simulink model "Hybrid_P2_Parallel_ETE"  (R2017b)
settings: Solver=FixedStepAuto  StartTime=0.0  StopTime=length(Speed)  FixedStep=0.01  MaxStep=0.01  RelTol=1e-3  EnableMultiTasking=on
PostLoadFcn:
  | , if any(exist('dsrtsu_mdlpostloadfcn', 'file') == [2, 3, 6]), try dsrtsu_mdlpostloadfcn('Execute', bdroot); catch fprintf('Error in PostLoadFcn (dsrtsu_mdlpostloadfcn) for model "%s":\n %s\n', bdroot, lasterr); end, end,
undefined symbols (not defined in the file): Actuators, APP1_OOR, APP2_OOR, APP_Mismatch, Brk_Flt, cal, ClutchEngag, CycLength, CycNmb, DiscIntNeverNeededParam, eng, Engine, EngOverTemp, ENGTRQ_MSMCH_Degraded_CP, ENGTRQ_MSMCH_ErrCritical_CP, ENGTRQ_MSMCH_LimpHome_CP, EngTrqMismatch, ess, ESSOverTemp, gb, Gearbox, KeyPos_Flt, lib_Actuators, lib_EMachine_2017a, lib_Sensors_2017a, Loss, LossCAN, Machine, MCUOverTemp, mot, MotDirMismatch, MotOverTemp, MotTrqMismatch, PRNDL_Flt, Ratio, RegenFault, Scope_new, Scopes1, Sensors, Spd, StopIndex, t_amb, time, tloop
libraries: simulink x117, EC2_libraries x9, powerlib_meascontrol x2, CalculationGallon x1, lib_Chassis x1, lib_DCDC x1, lib_Differential x1, lib_HVESS x1, lib_Engine x1, lib_OBC x1, lib_Transmission x1, Transmission_Validation x1
(part 9 of 10)

== system Hybrid_P2_Parallel_ETE/Controller_with_Transmission_Manager1/HSC/Powertrain Manager/HV Manager1/DCDC Manager/Override_Voltage ==
  In1 : Inport
  Switch : Switch  Criteria=u2 > Threshold
  VoltageHVOvrrdSW : Constant  Value=0
  voltageHVOvrrdVal : Constant  Value=0
  Out1 : Outport
  wires:
  voltageHVOvrrdVal/1 -> Switch/1
  VoltageHVOvrrdSW/1 -> Switch/2
  In1/1 -> Switch/3
  Switch/1 -> Out1/1  "DC_mode"

== system Hybrid_P2_Parallel_ETE/Controller_with_Transmission_Manager1/HSC/Powertrain Manager/HV Manager1/DCDC Manager/Override_VoltageLV ==
  In1 : Inport
  Switch : Switch  Criteria=u2 > Threshold
  VoltageLVOvrrdSW : Constant  Value=0
  VoltageLVOvrrdVAL : Constant  Value=14
  Out1 : Outport
  wires:
  VoltageLVOvrrdVAL/1 -> Switch/1
  VoltageLVOvrrdSW/1 -> Switch/2
  In1/1 -> Switch/3
  Switch/1 -> Out1/1  "DC_mode"

== system Hybrid_P2_Parallel_ETE/Controller_with_Transmission_Manager1/HSC/Powertrain Manager/HV Manager1/DCDC Manager/Override_mode ==
  In1 : Inport
  DCDCOVrrdSwitch : Constant  Value=0
  DCDCOVrrdVal : Constant  Value=0
  Switch : Switch  Criteria=u2 > Threshold
  Out1 : Outport
  wires:
  Switch/1 -> Out1/1  "DC_mode"
  In1/1 -> Switch/3
  DCDCOVrrdSwitch/1 -> Switch/2
  DCDCOVrrdVal/1 -> Switch/1

== system Hybrid_P2_Parallel_ETE/Controller_with_Transmission_Manager1/HSC/Powertrain Manager/Torque Distribution1/AxlTrq_to_EngTrq2/Ratio Filter ==
  Ratio : Inport
  Abs : Abs
  Compare To Zero : simulink/Logic and Bit Operations/Compare To Zero  relop===  OutDataTypeStr=boolean
  Constant : Constant  Value=cal.Time.TrnsOvrllEstTrqRatioSwitch
  Mature_Delay : EC2_libraries/Mature_Delay
  Memory1 : Memory  InitialCondition=1
  Switch1 : Switch  Threshold=1
  Switch2 : Switch  Threshold=1
  Filtered_Ratio : Outport
  wires:
  Ratio/1 -> Compare To Zero/1, Abs/1
  Compare To Zero/1 -> Mature_Delay/1, Switch2/2
  Abs/1 -> Switch1/1, Switch2/3
  Switch1/1 -> Switch2/1
  Constant/1 -> Mature_Delay/2
  Mature_Delay/1 -> Switch1/2
  Memory1/1 -> Switch1/3
  Switch2/1 -> Filtered_Ratio/1, Memory1/1  "gear_ratio"

== system Hybrid_P2_Parallel_ETE/Controller_with_Transmission_Manager1/HSC/Powertrain Manager/Torque Distribution1/AxlTrq_to_MotTrq/AxlTrq_to_MtrTrq2 ==
  note: //From motor axle torque to motor torque//
  In1 : Inport
  Compare To Constant : simulink/Logic and Bit Operations/Compare To Constant  relop===  const=0  OutDataTypeStr=boolean
  Constant1 : Constant  Value=max(gb.plant.init.ratio.map)
  Constant5 : Constant  Value=fd.plant.init.ratio
  Divide : Product  Inputs=*//
  Rate Limiter1 : RateLimiter  Commented=on  RisingSlewLimit=20000  FallingSlewLimit=-20000
  Ratio Filter : Subsystem
  Switch : Switch  Criteria=u2 > Threshold
  MtrTrqCmd : Outport
  wires:
  In1/1 -> Divide/1  "MotAxlTrq"
  Constant5/1 -> Divide/2
  [TransRatio] -> Ratio Filter/1(Ratio)
  Compare To Constant/1 -> Switch/2
  Constant1/1 -> Switch/1
  Divide/1 -> MtrTrqCmd/1  "Axl2MotTrq"
  Switch/1 -> Divide/3  "TrnsFilRatio"
  Ratio Filter/1(Filtered_Ratio) -> Switch/3, Compare To Constant/1  "FilteredRatio"

== system Hybrid_P2_Parallel_ETE/Controller_with_Transmission_Manager1/HSC/Powertrain Manager/Torque Distribution1/AxlTrq_to_MotTrq/electric machine filter ==
  trq : Inport
  Interval Test : simulink/Logic and Bit Operations/Interval Test  IntervalClosedRight=on  uplimit=0.02  IntervalClosedLeft=on  lowlimit=-0.02  OutDataTypeStr=boolean
  Switch : Switch  Threshold=0.5
  electric machine time response : TransferFcn  Denominator=[mot.plant.init.time_response 1]
  filtered : Outport
  wires:
  electric machine time response/1 -> Switch/3
  Interval Test/1 -> Switch/2
  trq/1 -> Interval Test/1, electric machine time response/1, Switch/1
  Switch/1 -> filtered/1  "MotTrqFil"

== system Hybrid_P2_Parallel_ETE/Controller_with_Transmission_Manager1/HSC/Powertrain Manager/Torque Distribution1/Hood_Status/Close_Voltage ==
  DC_Voltage : Inport
  Constant : Constant  Value=2.3
  Constant1 : Constant  Value=3.03
  Divide : Product  Inputs=*/*
  Out1 : Outport
  wires:
  Divide/1 -> Out1/1
  Constant/1 -> Divide/1
  Constant1/1 -> Divide/2
  DC_Voltage/1 -> Divide/3

== system Hybrid_P2_Parallel_ETE/Controller_with_Transmission_Manager1/HSC/Powertrain Manager/Torque Distribution1/Hood_Status/Open_Voltage ==
  DC_Voltage : Inport
  Constant2 : Constant  Value=0.73
  Constant3 : Constant  Value=3.03
  Divide1 : Product  Inputs=*/*
  Out1 : Outport
  wires:
  Divide1/1 -> Out1/1
  Constant2/1 -> Divide1/1
  DC_Voltage/1 -> Divide1/3
  Constant3/1 -> Divide1/2

== system Hybrid_P2_Parallel_ETE/Controller_with_Transmission_Manager1/HSC/Powertrain Manager/Torque Distribution1/IdealMotTrq/MotTrq2AxlTrq ==
  In1 : Inport
  Compare To Constant : simulink/Logic and Bit Operations/Compare To Constant  relop===  const=0  OutDataTypeStr=boolean
  Constant1 : Constant  Value=max(gb.plant.init.ratio.map)
  Constant2 : Constant  Value=fd.plant.init.ratio
  Divide1 : Product  Inputs=***
  Ratio Filter : Subsystem
  Switch : Switch  Criteria=u2 > Threshold
  Out1 : Outport
  wires:
  Ratio Filter/1(Filtered_Ratio) -> Compare To Constant/1, Switch/3  "FilteredRatio"
  Switch/1 -> Divide1/1  "TrnsFilRatio"
  Constant1/1 -> Switch/1
  Compare To Constant/1 -> Switch/2
  Constant2/1 -> Divide1/2
  [TransRatio] -> Ratio Filter/1(Ratio)
  In1/1 -> Divide1/3
  Divide1/1 -> Out1/1  "P"

== system Hybrid_P2_Parallel_ETE/Controller_with_Transmission_Manager1/HSC/Powertrain Manager/Torque Distribution1/IdealMotTrq/Subsystem ==
  Setpoint : Inport
  Actual : Inport  Port=2
  Add : Sum  Inputs=+-
  Add2 : Sum
  IdleTorqueVal : Constant  Value=7
  Kp : Constant  Value=0.2
  Product : Product
  Out1 : Outport
  wires:
  Actual/1 -> Add/2
  Setpoint/1 -> Add/1
  Kp/1 -> Product/2
  IdleTorqueVal/1 -> Add2/2
  Add2/1 -> Out1/1
  Add/1 -> Product/1
  Product/1 -> Add2/1

== system Hybrid_P2_Parallel_ETE/Controller_with_Transmission_Manager1/HSC/Powertrain Manager/Torque Distribution1/Supervisory  Control  Logic1/VehReady.CD_Mode.Drive_mode.MotTrqCalc2/Motor idle torque1 ==
  In1 : Inport
  Constant2 : Constant  Value=fd.plant.init.ratio
  Constant3 : Constant  Value=0
  Divide1 : Product  Inputs=***
  Out1 : Outport
  wires:
  In1/1 -> Divide1/1
  Constant2/1 -> Divide1/2
  Constant3/1 -> Divide1/3
  Divide1/1 -> Out1/1  "P"

== system Hybrid_P2_Parallel_ETE/Controller_with_Transmission_Manager1/HSC/Powertrain Manager/Torque Distribution1/Supervisory  Control  Logic1/VehReady.Eng_Charging_Stat.EngTrqCalc/Multiply by Zero fix ==
  In1 : Inport
  Compare To Constant : simulink/Logic and Bit Operations/Compare To Constant  relop===  const=0  OutDataTypeStr=boolean
  Constant5 : Constant  Value=max(gb.plant.init.ratio.map)
  Ratio Filter : Subsystem
  Switch : Switch  Criteria=u2 > Threshold
  Out1 : Outport
  wires:
  In1/1 -> Ratio Filter/1(Ratio)
  Compare To Constant/1 -> Switch/2
  Constant5/1 -> Switch/1
  Switch/1 -> Out1/1  "TrnsFilRatio"
  Ratio Filter/1(Filtered_Ratio) -> Switch/3, Compare To Constant/1  "FilteredRatio"

== system Hybrid_P2_Parallel_ETE/Camaro Plant Model/E-Machine/IMG Plant/Electric Machine/Thermal1/MotInv_loop/MCUOverTemp Fault ==
  In1 : Inport
  Gain : Gain  Gain=3
  Switch : Switch  Threshold=1
  Out1 : Outport
  wires:
  Switch/1 -> Out1/1
  Gain/1 -> Switch/1
  [MCUOverTemp] -> Switch/2
  In1/1 -> Gain/1, Switch/3

== system Hybrid_P2_Parallel_ETE/Camaro Plant Model/E-Machine/IMG Plant/Electric Machine/Thermal1/MotInv_loop/MotorOverTempFault ==
  In1 : Inport
  Gain : Gain  Gain=2
  Memory : Memory
  Switch1 : Switch  Threshold=1
  Out1 : Outport
  wires:
  Switch1/1 -> Out1/1
  Gain/1 -> Switch1/1
  [MotOverTemp] -> Switch1/2
  In1/1 -> Switch1/3, Memory/1
  Memory/1 -> Gain/1

== system Hybrid_P2_Parallel_ETE/Camaro Plant Model/E-Machine/IMG Plant/Electric Machine/Thermal1/Motor Thermal/Lower Limit ==
  In1 : Inport
  Constant3 : Constant  Value=Lolimit
  MinMax : MinMax  Function=max  Inputs=2
  Out1 : Outport
  wires:
  MinMax/1 -> Out1/1
  Constant3/1 -> MinMax/2
  In1/1 -> MinMax/1

== system Hybrid_P2_Parallel_ETE/Camaro Plant Model/E-Machine/Soft MCU/Torque Calculation1/max torque /Heat index/Divide ==
  note: Take care of
      | division by 0
  numerator : Inport
  denominator : Inport  Port=2
  Fcn : Fcn  Expr=u[1] / ( u[2] + eps*(u[2]==0) )
  Mux : Mux  Inputs=2
  quotient : Outport
  wires:
  denominator/1 -> Mux/2
  Fcn/1 -> quotient/1
  numerator/1 -> Mux/1
  Mux/1 -> Fcn/1

== system Hybrid_P2_Parallel_ETE/Camaro Plant Model/E-Machine/Soft MCU/Torque Calculation2/max torque /Heat index/Divide ==
  note: Take care of
      | division by 0
  numerator : Inport
  denominator : Inport  Port=2
  Fcn : Fcn  Expr=u[1] / ( u[2] + eps*(u[2]==0) )
  Mux : Mux  Inputs=2
  quotient : Outport
  wires:
  denominator/1 -> Mux/2
  Fcn/1 -> quotient/1
  numerator/1 -> Mux/1
  Mux/1 -> Fcn/1

== system Hybrid_P2_Parallel_ETE/Camaro Plant Model/Transmission/Transmission Plant/Gearbox/Speed Calculation/P//N/Subsystem2 ==
  In1 : Inport
  In2 : Inport  Port=2
  Fcn : Fcn  Expr=u[1]/(u[2]+eps)*(u[2]!=0)
  Mux : Mux  Inputs=2
  Out1 : Outport
  wires:
  In2/1 -> Mux/2
  Fcn/1 -> Out1/1
  In1/1 -> Mux/1
  Mux/1 -> Fcn/1

== system Hybrid_P2_Parallel_ETE/Camaro Plant Model/Transmission/Transmission Plant/Gearbox/Speed Calculation/P//N/input shaft free wheeling losses ==
  input shaft speed : Inport
  Constant1 : Constant  Value=0
  Fcn1 : Fcn  Expr=u==0
  Gain1 : Gain  Gain=0.15  SaturateOnIntegerOverflow=on  OutDataTypeStr=Inherit: Same as input  ParamDataTypeStr=Inherit: Same as input
  Switch2 : Switch  Threshold=0.5  SaturateOnIntegerOverflow=on  InputSameDT=on
  input shaft decel : Outport
  wires:
  Constant1/1 -> Switch2/1
  Switch2/1 -> Gain1/1
  Gain1/1 -> input shaft decel/1
  Fcn1/1 -> Switch2/2
  input shaft speed/1 -> Fcn1/1, Switch2/3

== system Hybrid_P2_Parallel_ETE/Camaro Plant Model/Transmission/Transmission Plant/Gearbox/Speed Calculation/R//D/S-R Flip-Flop ==
  S : Inport
  R : Inport  Port=2
  Demux : Demux  Outputs=2
  Logic : CombinatorialLogic  TruthTable=[0 1;0 1;1 0;0 1;1 0;0 1;1 0;1 0]
  Memory : Memory  InitialCondition=initial_condition  InheritSampleTime=on
  Mux : Mux  Inputs=3
  Q : Outport  InitialOutput=0
  !Q : Outport  Port=2  InitialOutput=1
  wires:
  Mux/1 -> Logic/1
  Logic/1 -> Demux/1
  Demux/2 -> !Q/1
  Demux/1 -> Q/1, Memory/1
  Memory/1 -> Mux/1
  S/1 -> Mux/2
  R/1 -> Mux/3

== system Hybrid_P2_Parallel_ETE/Controller_with_Transmission_Manager1/HSC/Camaro Fault Detection/Signal Diagnostic/ESS Signal Diagnostic/ESS SOC Validity Check/essSOCValidity_Check ==
  In1 : Inport
  Above Normal Operation : simulink/Logic and Bit Operations/Compare To Constant  relop===  const=3  OutDataTypeStr=boolean
  Below Normal Operation : simulink/Logic and Bit Operations/Compare To Constant  relop===  const=0  OutDataTypeStr=boolean
  Logical Operator : Logic  Operator=OR  AllPortsSameDT=off  OutDataTypeStr=boolean
  Logical Operator1 : Logic  Operator=NOT  AllPortsSameDT=off  OutDataTypeStr=boolean
  Out1 : Outport
  wires:
  In1/1 -> Above Normal Operation/1, Below Normal Operation/1
  Logical Operator/1 -> Logical Operator1/1
  Below Normal Operation/1 -> Logical Operator/1
  Above Normal Operation/1 -> Logical Operator/2
  Logical Operator1/1 -> Out1/1

== system Hybrid_P2_Parallel_ETE/Controller_with_Transmission_Manager1/HSC/Camaro Fault Detection/Signal Diagnostic/ESS Signal Diagnostic/ESS Temp Validity Check/essTsignalValidity_Check ==
  In1 : Inport
  Above Normal Operation : simulink/Logic and Bit Operations/Compare To Constant  relop===  const=4  OutDataTypeStr=boolean
  Below Normal Operation : simulink/Logic and Bit Operations/Compare To Constant  relop===  const=0  OutDataTypeStr=boolean
  Logical Operator : Logic  Operator=OR  AllPortsSameDT=off  OutDataTypeStr=boolean
  Logical Operator1 : Logic  Operator=NOT  AllPortsSameDT=off  OutDataTypeStr=boolean
  Out1 : Outport
  wires:
  Logical Operator1/1 -> Out1/1
  Above Normal Operation/1 -> Logical Operator/2
  Below Normal Operation/1 -> Logical Operator/1
  Logical Operator/1 -> Logical Operator1/1
  In1/1 -> Below Normal Operation/1, Above Normal Operation/1

== system Hybrid_P2_Parallel_ETE/Controller_with_Transmission_Manager1/HSC/Driver_Requests/APP_BPP to DrvIntndAxlTrq2/Post Driver Intnded Axle Torque/Brake Command/Latch ==
  Input : Inport
  Reset : Inport  Port=2
  Logical Operator1 : Logic  Operator=NOT  AllPortsSameDT=off  OutDataTypeStr=boolean
  Logical Operator2 : Logic  AllPortsSameDT=off  OutDataTypeStr=boolean
  Logical Operator3 : Logic  Operator=OR  AllPortsSameDT=off  OutDataTypeStr=boolean
  Memory1 : Memory
  Out1 : Outport
  wires:
  Logical Operator2/1 -> Logical Operator3/2
  Reset/1 -> Logical Operator1/1
  Memory1/1 -> Logical Operator2/2
  Logical Operator3/1 -> Out1/1, Memory1/1
  Logical Operator1/1 -> Logical Operator2/1
  Input/1 -> Logical Operator3/1

== system Hybrid_P2_Parallel_ETE/Controller_with_Transmission_Manager1/HSC/Driver_Requests/APP_BPP to DrvIntndAxlTrq2/Post Driver Intnded Axle Torque/Driver Intended Axle Torque/Ratio Filter ==
  Ratio : Inport
  Abs : Abs
  Compare To Zero : simulink/Logic and Bit Operations/Compare To Zero  relop===  OutDataTypeStr=boolean
  Constant : Constant  Value=cal.Time.TrnsOvrllEstTrqRatioSwitch
  Mature_Delay : EC2_libraries/Mature_Delay
  Memory1 : Memory  InitialCondition=1
  Switch1 : Switch  Threshold=1
  Switch2 : Switch  Threshold=1
  Filtered_Ratio : Outport
  wires:
  Ratio/1 -> Compare To Zero/1, Abs/1
  Compare To Zero/1 -> Mature_Delay/1, Switch2/2
  Abs/1 -> Switch1/1, Switch2/3
  Switch1/1 -> Switch2/1
  Constant/1 -> Mature_Delay/2
  Mature_Delay/1 -> Switch1/2
  Memory1/1 -> Switch1/3
  Switch2/1 -> Filtered_Ratio/1, Memory1/1  "gear_ratio"

== system Hybrid_P2_Parallel_ETE/Controller_with_Transmission_Manager1/HSC/Powertrain Manager/HV Manager1/BMS_Manager/Isolation Fault Calculation/Resistance_Measurement ==
  In1 : Inport
  In2 : Inport  Port=2
  Enable : EnablePort
  Add : Sum
  ISOfault : Constant
  ISOmultiplier : Constant  Value=256
  ISOnofault : Constant  Value=0
  Minimum Allowed Isolation Resistance : Switch  Criteria=u2 > Threshold  Threshold=500000
  Product : Product
  Product1 : Product
  Resistance Adjustment : Constant  Value=1000
  IsoFault : Outport
  wires:
  Minimum Allowed Isolation Resistance/1 -> IsoFault/1  "IsoFault"
  ISOnofault/1 -> Minimum Allowed Isolation Resistance/1
  Resistance Adjustment/1 -> Product1/2
  Product1/1 -> Minimum Allowed Isolation Resistance/2
  ISOfault/1 -> Minimum Allowed Isolation Resistance/3
  Add/1 -> Product1/1
  Product/1 -> Add/1
  In2/1 -> Add/2
  In1/1 -> Product/1
  ISOmultiplier/1 -> Product/2

== system Hybrid_P2_Parallel_ETE/Controller_with_Transmission_Manager1/HSC/Powertrain Manager/Torque Distribution1/AxlTrq_to_MotTrq/AxlTrq_to_MtrTrq2/Ratio Filter ==
  Ratio : Inport
  Abs : Abs
  Compare To Zero : simulink/Logic and Bit Operations/Compare To Zero  relop===  OutDataTypeStr=boolean
  Constant : Constant  Value=cal.Time.TrnsOvrllEstTrqRatioSwitch
  Mature_Delay : EC2_libraries/Mature_Delay
  Memory1 : Memory  InitialCondition=1
  Switch1 : Switch  Threshold=1
  Switch2 : Switch  Threshold=1
  Filtered_Ratio : Outport
  wires:
  Ratio/1 -> Compare To Zero/1, Abs/1
  Compare To Zero/1 -> Mature_Delay/1, Switch2/2
  Abs/1 -> Switch1/1, Switch2/3
  Switch1/1 -> Switch2/1
  Constant/1 -> Mature_Delay/2
  Mature_Delay/1 -> Switch1/2
  Memory1/1 -> Switch1/3
  Switch2/1 -> Filtered_Ratio/1, Memory1/1  "gear_ratio"

== system Hybrid_P2_Parallel_ETE/Controller_with_Transmission_Manager1/HSC/Powertrain Manager/Torque Distribution1/IdealMotTrq/MotTrq2AxlTrq/Ratio Filter ==
  Ratio : Inport
  Abs : Abs
  Compare To Zero : simulink/Logic and Bit Operations/Compare To Zero  relop===  OutDataTypeStr=boolean
  Constant : Constant  Value=cal.Time.TrnsOvrllEstTrqRatioSwitch
  Mature_Delay : EC2_libraries/Mature_Delay
  Memory1 : Memory  InitialCondition=1
  Switch1 : Switch  Threshold=1
  Switch2 : Switch  Threshold=1
  Filtered_Ratio : Outport
  wires:
  Switch2/1 -> Memory1/1, Filtered_Ratio/1  "gear_ratio"
  Memory1/1 -> Switch1/3
  Mature_Delay/1 -> Switch1/2
  Constant/1 -> Mature_Delay/2
  Switch1/1 -> Switch2/1
  Abs/1 -> Switch2/3, Switch1/1
  Compare To Zero/1 -> Switch2/2, Mature_Delay/1
  Ratio/1 -> Abs/1, Compare To Zero/1

== system Hybrid_P2_Parallel_ETE/Controller_with_Transmission_Manager1/HSC/Powertrain Manager/Torque Distribution1/Supervisory  Control  Logic1/VehReady.Eng_Charging_Stat.EngTrqCalc/Multiply by Zero fix/Ratio Filter ==
  Ratio : Inport
  Abs : Abs
  Compare To Zero : simulink/Logic and Bit Operations/Compare To Zero  relop===  OutDataTypeStr=boolean
  Constant : Constant  Value=cal.Time.TrnsOvrllEstTrqRatioSwitch
  Mature_Delay : Subsystem  AncestorBlock=EC2_libraries/Mature_Delay
  Memory1 : Memory  InitialCondition=1  InheritSampleTime=on
  Switch1 : Switch  Threshold=1
  Switch2 : Switch  Threshold=1
  Filtered_Ratio : Outport
  wires:
  Ratio/1 -> Compare To Zero/1, Abs/1
  Compare To Zero/1 -> Mature_Delay/1(In), Switch2/2
  Abs/1 -> Switch1/1, Switch2/3
  Switch1/1 -> Switch2/1
  Constant/1 -> Mature_Delay/2(MatTime)
  Mature_Delay/1(Out) -> Switch1/2
  Memory1/1 -> Switch1/3
  Switch2/1 -> Filtered_Ratio/1, Memory1/1  "gear_ratio"

== system Hybrid_P2_Parallel_ETE/Controller_with_Transmission_Manager1/HSC/Powertrain Manager/Torque Distribution1/Supervisory  Control  Logic1/VehReady.Eng_Charging_Stat.EngTrqCalc/Multiply by Zero fix/Ratio Filter/Mature_Delay ==
  In : Inport
  MatTime : Inport  Port=2
  Gain : Gain  Gain=-1
  Lower Limit : EC2_libraries/Lower Limit  Lolimit=0.001
  Memory1 : Memory  InheritSampleTime=on
  Relational Operator1 : RelationalOperator  Operator=>  OutDataTypeStr=boolean  RndMeth=Nearest
  StepTm[sec] : Constant  Value=tloop
  Sum : Sum  Inputs=|++
  Switch1 : Switch  Threshold=1
  Out : Outport
  wires:
  Lower Limit/1 -> Relational Operator1/1
  Sum/1 -> Lower Limit/1, Memory1/1
  Switch1/1 -> Sum/1
  StepTm[sec]/1 -> Switch1/1
  MatTime/1 -> Relational Operator1/2
  Relational Operator1/1 -> Out/1
  Memory1/1 -> Gain/1, Sum/2
  Gain/1 -> Switch1/3
  In/1 -> Switch1/2

== matlab function Hybrid_P2_Parallel_ETE/Camaro Plant Model/E-Machine/Soft MCU/diff_INV_state ==
  data: u input; y output
function y = fcn(u)
if(u == 3) %when inverter is in standby state
    y = 0;
elseif(u == 8) %when inverter is in torque control state
    y = 1;
elseif(u==14) %when invertor is in error state
    y = 2;
else
    y = 0;
end

== stateflow chart Hybrid_P2_Parallel_ETE/Controller_with_Transmission_Manager1/HSC/Powertrain Manager/HV Manager1/DCDC Manager/Chart ==
  state Init
    en:
    DCDC_State = 1;
  state Power_On
    entry: DCmode = 1;
    DCDC_State = 2;
    VoltageHV = 0;
    VoltageLV =14;
    CurrentHV = 20;
    CurrentLV = 173;
  state Delay
    en:
    DCDC_State =2.5;
  state DCDC_Off
    entry: DCDC_State = 3;
    DCmode = 0;
  (default) -> Init
  Init -> Power_On : [ContactorsFailed == 0]
  Delay -> Power_On : after(3,sec)
      | [ContactorsFailed == 0]
  Power_On -> DCDC_Off : [CloseMainC == 0 || INV_state == 14 || ContactorsFailed == 1]
  DCDC_Off -> Delay : [(INV_state == 3 || INV_state == 8)&& (powerMode ==1|| powerMode == 2 || powerMode == 3)]
  data: BMS_IstModus input; CloseMainC input; DCmode output; VoltageHV output; CurrentHV output; VoltageLV output; CurrentLV output; INV_state input; DCDC_State output; EngOnReq input; powerMode input; mode input; keypos input; Contactor local; ContactorsFailed input

== stateflow chart Hybrid_P2_Parallel_ETE/Controller_with_Transmission_Manager1/HSC/Camaro Fault Detection/Component Diagnostic/Driver Input Diagnostic/Driver_Input_Diag ==
  state Driver_Input_Offline
    en: Driver_Input_Status=0;
  state Driver_Input_Online
    en: Driver_Input_Status=1;
  (default) -> Driver_Input_Offline
  Driver_Input_Online -> Driver_Input_Offline : [~APP_Valid|| ~Drv_BPP_SigValid||~KeyPos||~PRNDL||BrakeFail]
  Driver_Input_Offline -> Driver_Input_Online : [APP_Valid&&Drv_BPP_SigValid&&KeyPos&&PRNDL&&BrakeFail==0]
  data: APP_Valid input; Drv_BPP_SigValid input; KeyPos input; Driver_Input_Status output; PRNDL input; BrakeFail input

== stateflow chart Hybrid_P2_Parallel_ETE/Controller_with_Transmission_Manager1/HSC/Powertrain Manager/Torque Distribution1/EngineCharge Logic ==
  state EngineChg
    entry:
    CDmodeSW=0;
  state Hybrid_Mode
    entry:
    CDmodeSW=1;
  Hybrid_Mode -> EngineChg : [(SW_Engine_On==1&&SW_CS_On ==0)|| (SW_Engine_On == 0 && SW_CS_On == 1)]
  (default) -> Hybrid_Mode
  EngineChg -> Hybrid_Mode : [SW_Engine_On==0 && SW_CS_On==0]
  data: SW_Engine_On input; CDmodeSW output; SW_CS_On input

== stateflow chart Hybrid_P2_Parallel_ETE/Controller_with_Transmission_Manager1/HSC/Camaro Fault Detection/Component Diagnostic/ESS Component Diagnostic/BMS_CompDiag1 ==
  state BMS_Offline
    en: BMS_Status=0;
  state BMS_Online
    en:BMS_Status=2;
  state BMS_Limited
    en: BMS_Status=1;
  BMS_Offline -> BMS_Online [order 1] : [BMS_RollingAliveActive_SigValid&&BMS_contactorsFailed_SigValid&&...
      | BMS_essTemp_SigValid&&ClearFault&&BMS_essSOC_0_1_SigValid&&...
      | ess_GroundFault&&essCur_A_SigValid]
  (default) -> BMS_Offline
  BMS_Online -> BMS_Offline [order 2] : [~BMS_RollingAliveActive_SigValid||...
      | ~BMS_contactorsFailed_SigValid||~BMS_essSOC_0_1_SigValid|| ...
      | ~ess_GroundFault]
  BMS_Limited -> BMS_Offline [order 2] : [~BMS_RollingAliveActive_SigValid||...
      | ~BMS_contactorsFailed_SigValid]
  BMS_Offline -> BMS_Limited [order 2] : [BMS_RollingAliveActive_SigValid &&...
      | BMS_contactorsFailed_SigValid && ~BMS_essTemp_SigValid||...
      |  ~BMS_essSOC_0_1_SigValid]
  BMS_Limited -> BMS_Online [order 1] : [BMS_essTemp_SigValid||...
      | ClearFault||BMS_essSOC_0_1_SigValid]
  BMS_Online -> BMS_Limited [order 1] : [~BMS_essTemp_SigValid||...
      |  ~BMS_essSOC_0_1_SigValid]
  data: BMS_RollingAliveActive_SigValid input; BMS_contactorsFailed_SigValid input; BMS_essTemp_SigValid input; BMS_Status output; BMS_essSOC_0_1_SigValid input; essCur_A_SigValid input; ess_GroundFault input; ClearFault input

== stateflow chart Hybrid_P2_Parallel_ETE/Controller_with_Transmission_Manager1/HSC/Camaro Fault Detection/Component Diagnostic/Engine Component Diagnostic/ECM_CompDiag ==
  state ECM_Offline
    en: ECM_Status=0;
  state ECM_Online
    en:ECM_Status=2;
  state ECM_Limited
    en: ECM_Status=1;
  ECM_Online -> ECM_Offline [order 2] : [~ECM_RollingAliveActive||~engTrqCmdRecvd_SigValid||...
      | ~Engine_Speed_rpm_SigValid||Eng_TempRange_123==3||Eng_Torq_Msmch==1||ClearFault==0]
  (default) -> ECM_Offline
  ECM_Offline -> ECM_Online [order 1] : [ECM_RollingAliveActive&&engTrqCmdRecvd_SigValid &&...
      | Engine_Speed_rpm_SigValid&&ClearFault&&Eng_TempRange_123==1&&Eng_Torq_Msmch==0&&ClearFault]
  ECM_Limited -> ECM_Offline [order 2] : [~ECM_RollingAliveActive||~engTrqCmdRecvd_SigValid||~Engine_Speed_rpm_SigValid|| Eng_TempRange_123==3||Eng_Torq_Msmch==1]
  ECM_Offline -> ECM_Limited [order 2] : [ECM_RollingAliveActive...
      | &&engTrqCmdRecvd_SigValid &&Engine_Speed_rpm_SigValid...
      | &&Eng_Torq_Msmch==0&&[Eng_TempRange_123==2 ]]
  ECM_Online -> ECM_Limited [order 1] : [ECM_RollingAliveActive...
      | &&engTrqCmdRecvd_SigValid &&Engine_Speed_rpm_SigValid...
      | &&Eng_Torq_Msmch==0&&(Eng_TempRange_123==2 )]
  ECM_Limited -> ECM_Online [order 1] : [Eng_TempRange_123==1&&Eng_Torq_Msmch==0]
  data: ECM_RollingAliveActive input; engTrqCmdRecvd_SigValid input; Eng_Torq_Msmch input; Engine_Speed_rpm_SigValid input; Eng_TempRange_123 input; ECM_Status output; ClearFault input

== stateflow chart Hybrid_P2_Parallel_ETE/Controller_with_Transmission_Manager1/HSC/Camaro Fault Detection/Component Diagnostic/Engine Component Diagnostic/Eng_Torq_MsmchLevel ==
  state Normal_Torque
    en: Eng_Torq_MsmchLevel==1
  state Creep_Torq_Allowed
    en: Eng_Torq_MsmchLvel==3
  state AboveMax
    en: Eng_Torq_MsmchLevel==4
  state Max_power_limited
    en: Eng_Torq_MsmchLvel==2
  (default) -> Normal_Torque
  AboveMax -> Normal_Torque [order 2] : [SignalValue<ENGTRQ_MSMCH_Degraded_CP]
  Creep_Torq_Allowed -> AboveMax [order 2] : [SignalValue>ENGTRQ_MSMCH_ErrCritical_CP]
  Max_power_limited -> Normal_Torque [order 1] : [SignalValue<ENGTRQ_MSMCH_Degraded_CP]
  Normal_Torque -> Max_power_limited [order 1] : [SignalValue>ENGTRQ_MSMCH_Degraded_CP&&...
      | SignalValue<ENGTRQ_MSMCH_LimpHome_CP]
  Normal_Torque -> AboveMax [order 2] : [SignalValue>ENGTRQ_MSMCH_ErrCritical_CP]
  AboveMax -> Creep_Torq_Allowed [order 1] : [SignalValue>ENGTRQ_MSMCH_LimpHome_CP&&SignalValue<ENGTRQ_MSMCH_ErrCritical_CP]
  Creep_Torq_Allowed -> Max_power_limited [order 1] : [SignalValue<ENGTRQ_MSMCH_LimpHome_CP&&SignalValue>ENGTRQ_MSMCH_Degraded_CP]
  Max_power_limited -> Creep_Torq_Allowed [order 2] : [SignalValue>ENGTRQ_MSMCH_LimpHome_CP&&SignalValue<ENGTRQ_MSMCH_ErrCritical_CP]
  data: SignalValue input; ENGTRQ_MSMCH_Degraded_CP parameter; ENGTRQ_MSMCH_LimpHome_CP parameter; Eng_Torq_MsmchLevel output; ENGTRQ_MSMCH_ErrCritical_CP parameter

== stateflow chart Hybrid_P2_Parallel_ETE/Controller_with_Transmission_Manager1/HSC/Camaro Fault Detection/Signal Diagnostic/Driver Signal Diagnostic/AccPedalValidity ==
  state SignalHigh
    en: signalValid=0;
  state SignalInRange
  state SignalLow
    en:signalValid=0;
  SignalHigh -> SignalInRange : [signalValue<=100]
  SignalInRange -> SignalHigh [order 1] : [signalValue>102]
  SignalInRange -> SignalInRange [order 3] : [clearFaults==1]
      | {signalValid=1;}
  (default) -> SignalInRange : {signalValid=1;}
  SignalLow -> SignalInRange : [signalValue>0]
  SignalInRange -> SignalLow [order 2] : [signalValue<-0.5]
  data: clearFaults input; signalValue input; signalValid output

== stateflow chart Hybrid_P2_Parallel_ETE/Controller_with_Transmission_Manager1/HSC/Powertrain Manager/HV Manager1/BMS_Manager/ESS_Manager ==
  state Ground_Fault
    entry:
    HV_State=-8;
    GFD_Light=1
  state Fault_light_OFF
    entry: GFD_Light=0;
    HV_State=-9;
  state Voltage_Fault
    en:
    HV_State=-11;
  state HVIL_Fault
    entry: MO_BMS_Sollmodus=0;
    HV_State=-10;
  state HV_Startup
    state BMS_Wake
      entry:  HV_State=1;
      T_15=1;
      MO_BMS_Sollmodus=0;
      HVDischarge=0;
    state Clear_Faults
      entry:
      Diag_Rq_Fktnl_Data_OBD_byte_0 =1;
      Diag_Rq_Fktnl_Data_OBD_byte_1=4;
      Diag_Rq_Fktnl_Data_OBD_byte_2=0;
      Diag_Rq_Fktnl_Data_OBD_byte_3=0;
      Diag_Rq_Fktnl_Data_OBD_byte_4=0;
      Diag_Rq_Fktnl_Data_OBD_byte_5=0;
      Diag_Rq_Fktnl_Data_OBD_byte_6=0;
      Diag_Rq_Fktnl_Data_OBD_byte_7=0;
      HV_State=2;
    state Charge_Wake
      entry: chga_wake=1;
      HV_State=3;
    state Drive_Wake
      entry: veh_wake=1;
      HV_State=8;
    state BMS_Enable_Charge
      entry: MO_BMS_Sollmodus=0;
      HV_State=4;
    state BMS_Enable_Drive
      entry: MO_BMS_Sollmodus=0;
      HV_State=9;
    state Power_Contactors_Drive
      en:
      MO_BMS_Sollmodus=0;
      T_30C = 1;
      HV_State=10;
    state Power_Contactors_Charge
      en: MO_BMS_Sollmodus=0;
      T_30C = 1;
      HV_State=5;
    state Close_Contactors_Drive
      entry:
      MO_BMS_Sollmodus=1;
      HV_State=11;
    state Close_Contactors_Charge
      entry:
      MO_BMS_Sollmodus=1;
      HV_State=6;
    state Time_delay
    state Ready_to_Charge
      entry: ReadyToCharge=1;
      ISO_Hybrid_01_Req = 1;
      HV_State=7;
    state Ready_to_Drive
      entry: ReadyToDrive=1;
      ISO_Hybrid_01_Req = 1;
      HV_State=12;
    (default) -> BMS_Wake
    BMS_Wake -> Clear_Faults : after(0.1,sec)
    Clear_Faults -> Charge_Wake [order 1] : [plugged]
    Clear_Faults -> Drive_Wake [order 2] : after(0.15,sec)
    Drive_Wake -> BMS_Enable_Drive : [BMS_Fehler_Pilot==0 ]
    Charge_Wake -> BMS_Enable_Charge : [BMS_Fehler_Pilot==0 ]
    BMS_Enable_Charge -> Power_Contactors_Charge : [BMS_Init_abgeschlossen]
    BMS_Enable_Drive -> Power_Contactors_Drive : [BMS_Init_abgeschlossen]
    Power_Contactors_Drive -> Close_Contactors_Drive : [closeMaincReq]
    Power_Contactors_Charge -> Close_Contactors_Charge : [closeMaincReq]
    Close_Contactors_Charge -> Time_delay : [BMS_Fehler_HS_offen==0&&(BMS_IstModus==4||BMS_IstModus==1)]
    Close_Contactors_Drive -> Ready_to_Drive : [BMS_Fehler_HS_offen==0&&BMS_IstModus==1]
    Time_delay -> Ready_to_Charge : after(1,sec)
    Ready_to_Drive -> Ready_to_Charge : [plugged]
    Ready_to_Charge -> Ready_to_Drive : [plugged==0]
  note: // Rev 2_14_2017
      | Added plugged to Off-On transition
      | Added EnableInverter to charge path
      | Changed IstModus to 1 at the end of charge path
      |
      | Create HV On Request block to request charging when vehicle is off
  state HV_Shudown
    state MCU_Delay
      en:
      HV_State = -1;
    state Open_Contactors
      entry: MO_BMS_Sollmodus=0;
      HV_State=-2;
      ISO_Hybrid_01_Req = 0;
    state ShutDown_T30C
      entry: T_30C=0;
    state Discharge_Bus
      entry: HVDischarge=1;
      HV_State=-3;
    state Disable_BCM_1
      entry: T_15=0;
      HVDischarge=0;
      HV_State=-4;
    state Disable_BCM_2
      entry: T_30=0;
      HVDischarge=0;
      HV_State=-5;
    state Send_BCM_to_Sleep
      en: MO_SleepAckn =1;
      T_15=0;
      T_30=0;
      HV_State=-6;
    state Shutdown_Complete
      entry: Shutdown_Complete=1;
      HV_State=-7;
    (default) -> MCU_Delay
    MCU_Delay -> Open_Contactors : [MCU_State >= 9]
    Open_Contactors -> ShutDown_T30C : after(2,sec)
    ShutDown_T30C -> Discharge_Bus : [BMS_IstModus==5]
    Discharge_Bus -> Disable_BCM_1 : [BMS_Spannung_ZwKr<30]
    Disable_BCM_1 -> Disable_BCM_2 : [BMS_IstStrom<0.02]
    Disable_BCM_2 -> Send_BCM_to_Sleep
    Send_BCM_to_Sleep -> Shutdown_Complete : [BMS_SleepInd]
  note: //Rev 8_21_2017
      | //Removed all engine related conditions
      | //Removed EngRunATV
  Voltage_Fault -> HV_Shudown : after(0.25, sec)
  Ground_Fault -> Fault_light_OFF : [(ISOfault==0&&KeyPos==1)||(ISOfault==0&&KeyPos==0&&plugged==1)]
  HV_Shudown -> Ground_Fault [order 2] : [ISOfault==1]
  Fault_light_OFF -> HV_Shudown
  HV_Startup -> Ground_Fault [order 3] : [ISOfault==1]
  HV_Startup -> HVIL_Fault [order 4] : [BMS_Fehler_Pilot]
  HVIL_Fault -> HV_Shudown : [BMS_Fehler_Pilot==0]
  HV_Startup -> Voltage_Fault [order 1] : after(5,sec)
      | [BMS_Spannung_ZwKr<50&&EngRunAtv]
  (default) -> HV_Shudown
  HV_Shudown -> HV_Startup [order 1] : [HV_req==1||plugged||EngRunAtv]
  HV_Startup -> HV_Shudown [order 2] : [(HV_req==0 && plugged==0) || SoC < 10]
      | {ReadyToDrive = 0;
      | ReadyToCharge = 0;}
  data: data local; ISOfault input; plugged input; BMS_Fehler_HS_offen input; BMS_Fehler_Pilot input; BMS_Init_abgeschlossen input; BMS_IstModus input; BMS_IstSpannung input; BMS_IstStrom input; BMS_SleepInd input; Diag_Rq_Fktnl_Data_OBD_byte_0 output; Diag_Rq_Fktnl_Data_OBD_byte_1 output; Diag_Rq_Fktnl_Data_OBD_byte_2 output; Diag_Rq_Fktnl_Data_OBD_byte_3 output; Diag_Rq_Fktnl_Data_OBD_byte_4 output; Diag_Rq_Fktnl_Data_OBD_byte_5 output; Diag_Rq_Fktnl_Data_OBD_byte_6 output; Diag_Rq_Fktnl_Data_OBD_byte_7 output; ISO_Hybrid_01_Req output; MO_SleepAckn output; MO_BMS_Sollmodus output; T_15 output; T_30 output; T_30C output; veh_wake output; chga_wake output; HVDischarge output; HV_State output; ReadyToDrive output; ReadyToCharge output; Shutdown_Complete output; HV_req input boolean; BMS_Spannung_ZwKr input; NMH_BMS_Car_WakeUp input; NMH_Normal_Mode_1 input; NMH_BMS_Normal_Mode_2 input; NMH_BMS_Start_1 input; NMH_BMS_Start_2 input; timer local; KeyPos input; GFD_Light output; EngRunAtv input; closeMaincReq input boolean; INV_State input; SoC input; MCU_State input

== stateflow chart Hybrid_P2_Parallel_ETE/Controller_with_Transmission_Manager1/HSC/Camaro Fault Detection/Signal Diagnostic/Driver Signal Diagnostic/AccPedalValidity1 ==
  state SignalHigh
    en: signalValid=0;
  state SignalInRange
  state SignalLow
    en:signalValid=0;
  SignalHigh -> SignalInRange : [signalValue<=100]
  SignalInRange -> SignalHigh [order 1] : [signalValue>102]
  SignalInRange -> SignalInRange [order 3] : [clearFaults==1]
      | {signalValid=1;}
  (default) -> SignalInRange : {signalValid=1;}
  SignalLow -> SignalInRange : [signalValue>0]
  SignalInRange -> SignalLow [order 2] : [signalValue<-0.5]
  data: clearFaults input; signalValue input; signalValid output

== stateflow chart Hybrid_P2_Parallel_ETE/Controller_with_Transmission_Manager1/HSC/Camaro Fault Detection/Signal Diagnostic/Driver Signal Diagnostic/BrakeFailureDetection/Chart ==
  state No_Fault
    en:
    DecelFail=0;
  state Detection_State
    en:
    Detection_state=1;
  state No_Fault1
    en:
    DecelFail=0;
  state Detection_State1
    en:
    Detection_state=2;
  state No_Fault2
    en:
    DecelFail=0;
  state Detection_State2
    en:
    Detection_state=3;
    du:
    DecelFail=1;
  (default) -> (junction 3)
  (junction 3) -> No_Fault [order 2]
  (junction 3) -> Detection_State [order 1] : [VehSpeed>0]
  Detection_State -> (junction 8)
  (junction 8) -> No_Fault1 [order 2]
  (junction 8) -> Detection_State1 [order 1] : [BPP>0]
  Detection_State1 -> (junction 15)
  (junction 15) -> No_Fault2 [order 2]
  (junction 15) -> Detection_State2 [order 1] : [Incre||Unchange]
  data: BPP input; VehSpeed input; Incre input; Unchange input; DecelFail output; Detection_state local

== stateflow chart Hybrid_P2_Parallel_ETE/Controller_with_Transmission_Manager1/HSC/Powertrain Manager/HV Manager1/Inverter Manager/MCU_Manager  ==
  state MCU_Initialization
    state MCU_Request_Standby
      en:
      MCU_State = 1;
      RequestedStateINV = 3;
      CAN_Activation = 1;
    state Power_Off_INVCON
      entry:
      MCU_State = 0;
      INVCON_Power =0;
    state Power_On_INVCON
      en:MCU_State = 2;
      INVCON_Power =1;
    state HV_CAN_Actuation_Fault
      en:
      MCU_State = -1;
      CAN_Activation = 0;
    state INVCON_Power_Fault
      en:
      MCU_State = -2;
      INVCON_Power =0;
      CAN_Activation = 0;
    Power_Off_INVCON -> (junction 18) : {Timer=0;}
    (junction 18) -> MCU_Request_Standby [order 1] : [HVCAN_State]
    HV_CAN_Actuation_Fault -> (junction 18) : [HVCAN_State]
    (junction 18) -> HV_CAN_Actuation_Fault [order 2] : after(3,sec)
    (default) -> Power_Off_INVCON
    MCU_Request_Standby -> Power_On_INVCON : [HV_State == 9]
    Power_On_INVCON -> INVCON_Power_Fault : after(3,sec)
        | [INV_State ~= 3]
  state MCU_TorqueMode
    state MCU_Enable
      en:MCU_State = 4;
      RequestedStateINV = 8;
      during: Timer = Timer + 1;
    state MCU_Ready
      en:
      MCU_State = 3;
    state MCU_Running
      en:
      MCU_State =5;
    state TorqueCommand_Reject_Fault
      en:
      MCU_State = -3;
      RequestedStateINV = 3;
    state MCU_Stop
      en:
      MCU_State = 6;
      RequestedStateINV = 3;
    (default) -> MCU_Ready
    MCU_Enable -> (junction 35)
    (junction 35) -> MCU_Running [order 1] : [INV_State == 8]
    MCU_Ready -> MCU_Enable : [EnableInverter]
        | {Timer = 0;}
    (junction 35) -> TorqueCommand_Reject_Fault [order 2] : after(10,sec)
    MCU_Running -> MCU_Stop : [~ReadyToDrive]
  state MCU_Shutdown
    state MCU_Off
      en:
      MCU_State = 11;
      RequestedStateINV = 3;
      INVCON_Power = 0;
    state MCU_Dschrg
      en:
      MCU_State = 10;
      RequestedStateINV = 14;
    state MCU_RdyForShtDwn
      en:
      MCU_State = 9;
    (default) -> MCU_RdyForShtDwn
    MCU_RdyForShtDwn -> MCU_Dschrg : [~EnableInverter]
        | {Timer = 0;}
    MCU_Dschrg -> MCU_Off : [INV_State == 14 && LinkVoltage<60]
  (default) -> MCU_Initialization
  MCU_Shutdown -> MCU_Initialization : [KeyPos>= 1]
  MCU_Initialization -> MCU_Shutdown [order 2] : [ReadyToCharge]
  MCU_TorqueMode -> MCU_Initialization [order 1] : [INV_State == 14]
  MCU_Initialization -> MCU_TorqueMode [order 1] : [INV_State == 3 && INVCON_Power_Feedback && ReadyToDrive]
  MCU_TorqueMode -> MCU_Shutdown [order 2] : [INV_State == 3 && ~ReadyToDrive]
  data: ReadyToDrive input boolean; ReadyToCharge input; HV_State input; HVCAN_State input boolean; INVCON_Power_Feedback input; KeyPos input; LinkVoltage input; INV_State input; INV_CurrentHV input; Timer local double; MCU_State output; EnableInverter input boolean; ShutdownCurrent input; INVCON_Power output double; RequestedStateINV output; CAN_Activation output

== matlab function Hybrid_P2_Parallel_ETE/Camaro Plant Model/E-Machine/Soft MCU/diff_INV_state1 ==
  data: u input; y output
function y = fcn(u)
if(u == 0) %when inverter is in standby state
    y = 0;
elseif(u == 1) %when inverter is in torque control state
    y = 1;
elseif(u==2) %when invertor is in error state
    y = 0;
else
    y = 0;
end

== stateflow chart Hybrid_P2_Parallel_ETE/Controller_with_Transmission_Manager1/HSC/Powertrain Manager/Torque Distribution1/Hood_Status/Hood Status ==
  state Hood_Closed
    du:
    Hood_Status=0;
  state Hood_Open
    du:
    Hood_Status=1;
  Hood_Open -> Hood_Closed : [HoodSig_Voltage<=HoodCloseVolt+1.5&&...
      | HoodSig_Voltage>=HoodCloseVolt-1.5]
  (default) -> Hood_Open
  Hood_Closed -> Hood_Open : [HoodSig_Voltage<=HoodOpenVolt+1.5&&...
      | HoodSig_Voltage>=HoodOpenVolt-1.5]
  data: HoodCloseVolt input; HoodOpenVolt input; Hood_Status output; HoodSig_Voltage input

== stateflow chart Hybrid_P2_Parallel_ETE/Controller_with_Transmission_Manager1/HSC/Camaro Fault Detection/Signal Diagnostic/ESS Signal Diagnostic/ESS SOC Validity Check/essSOC_0_1Range ==
  state aboveMax
    en: essSOCRange=3;
  state NormalRange
    en: essSOCRange=2;
  state LowRange
    en:essSOCRange=1;
  state BelowNormal
    en: essSOCRange=0;
  aboveMax -> NormalRange : [signalValue<0.95]
  NormalRange -> aboveMax [order 1] : [signalValue>=0.95]
  NormalRange -> NormalRange [order 3] : [clearFaults==1]
      | {essSOCRange=2;}
  (default) -> NormalRange
  LowRange -> NormalRange [order 1] : [signalValue>0.3]
  NormalRange -> LowRange [order 2] : [signalValue<=0.3&&signalValue>0.15]
  LowRange -> BelowNormal [order 2] : [signalValue<=0.15]
  BelowNormal -> LowRange : [signalValue>0.15]
  data: clearFaults input; signalValue input; data local; essSOCRange output

== stateflow chart Hybrid_P2_Parallel_ETE/Controller_with_Transmission_Manager1/HSC/Camaro Fault Detection/Signal Diagnostic/ESS Signal Diagnostic/ESS Temp Validity Check/essTsignalRange ==
  state AboveMax
    en: essTempRange=4;
  state HighRange
    en: essTempRange=3;
  state NormalRange
    en: essTempRange=2;
  state LowRange
    en:essTempRange=1;
  state BelowNormal
    en: essTempRange=0;
  HighRange -> AboveMax [order 2] : [signalValue>55]
  AboveMax -> HighRange : [signalValue<55]
  HighRange -> NormalRange [order 1] : [signalValue<=30]
  NormalRange -> HighRange [order 1] : [signalValue>32]
  NormalRange -> NormalRange [order 3] : [clearFaults==1]
      | {essTempRange=2;}
  (default) -> NormalRange
  LowRange -> NormalRange [order 1] : [signalValue>=30]
  NormalRange -> LowRange [order 2] : [signalValue<0 ]
  LowRange -> BelowNormal [order 2] : [signalValue<-28]
  BelowNormal -> LowRange : [signalValue>28]
  data: clearFaults input; signalValue input; essTempRange output; data local

== stateflow chart Hybrid_P2_Parallel_ETE/Controller_with_Transmission_Manager1/HSC/Camaro Fault Detection/Signal Diagnostic/ESS Signal Diagnostic/Rolling Alive Counter Detection/Chart ==
  state Off
    en:flag=0;
  state Alive
    en:flag=1;
  state Dead
    en:flag=0;
  Alive -> Alive [order 1] : after(CycleTime-tloop,sec)
      | [PulseDetect==1]
  (default) -> Off
  Off -> Alive : [PulseDetect==1]
  Alive -> Dead [order 2] : after(CycleTime,sec)
  data: PulseDetect input; CycleTime input; flag output; tloop input

== stateflow chart Hybrid_P2_Parallel_ETE/Controller_with_Transmission_Manager1/HSC/Camaro Fault Detection/Signal Diagnostic/Engine Signal Diagnostic/Rolling Alive Counter Detection1/Chart ==
  state Off
    en:flag=0;
  state Alive
    en:flag=1;
  state Dead
    en:flag=0;
  Alive -> Alive [order 1] : after(CycleTime-tloop,sec)
      | [PulseDetect==1]
  (default) -> Off
  Off -> Alive : [PulseDetect==1]
  Alive -> Dead [order 2] : after(CycleTime,sec)
  data: PulseDetect input; CycleTime input; flag output; tloop parameter

== stateflow chart Hybrid_P2_Parallel_ETE/Controller_with_Transmission_Manager1/HSC/Camaro Fault Detection/Signal Diagnostic/Transmission Signal Diagnostic/Rolling Alive Counter Detection/Chart ==
  state Off
    en:flag=0;
  state Alive
    en:flag=1;
  state Dead
    en:flag=0;
  Alive -> Alive [order 1] : after(CycleTime-tloop,sec)
      | [PulseDetect==1]
  (default) -> Off
  Off -> Alive : [PulseDetect==1]
  Alive -> Dead [order 2] : after(CycleTime,sec)
  data: PulseDetect input; CycleTime input; flag output; tloop parameter

== stateflow chart Hybrid_P2_Parallel_ETE/Camaro Plant Model/Transmission/Soft TCM/6L45 Logic ==
  settings: sampleTime=0.04
  state Torque_Converter_Control [parallel]
    du:
    du:[lockup_thrsh]=calc_lockup(Gear_D, drvAPP);
    du:[unlock_thrsh]=calc_unlock(Gear_D, drvAPP);
    settings: executionOrder=1
    state lockup_th = calc_lockup(Gear, APP) [function]
    note: Lever Position:
        | 1 P
        | 2 R
        | 3 N
        | 4 D
        |
        | 1 clutch lock-up
        | 0 clutch unlock
    state Lock
      en:
      LockupCmd = 1;
    state Unlock
      en:
      LockupCmd = 0;
    state unlock_th = calc_unlock(Gear,APP) [function]
    (default) -> Unlock
    Unlock -> Lock : [(Gear_D >= 4 || drvBPP > 0) && VehicleSpeed > 20]
    Lock -> Unlock : [VehicleSpeed < 20 || drvBPP == 0 && drvAPP > 5 && Gear_D <= 3]
  state Gearbox_Control [parallel]
    settings: executionOrder=2
    state Shifter_Actuator [parallel]
      settings: executionOrder=1
      state Shifter_D
        du:
        TransEstGear = Gear_D;
      state Shifter_R
        en:
        TransEstGear = 14;
      state Shifter_N
        en:
        TransEstGear = 13;
      state Shifter_P
        en:
        TransEstGear = 15;
      (default) -> Shifter_P
      Shifter_D -> Shifter_N : [ShftLvrPos <= 3]
      Shifter_N -> Shifter_R [order 2] : [ShftLvrPos <= 2]
      Shifter_R -> Shifter_P [order 2] : [ShftLvrPos <= 1]
      Shifter_N -> Shifter_D [order 1] : [ShftLvrPos >= 4]
      Shifter_R -> Shifter_N [order 1] : [ShftLvrPos >= 3]
      Shifter_P -> Shifter_R : [ShftLvrPos >= 2]
    state Shift_Schedule [parallel]
      settings: executionOrder=2
      state Gear_State_D [parallel]
        settings: executionOrder=1
        state Gear_4th
          entry:
          Gear_D = 4;
        state Gear_3rd
          entry:
          Gear_D = 3;
        state Gear_6th
          entry:
          Gear_D = 6;
        state Gear_7th
          entry:
          Gear_D = 7;
        state Gear_8th
          entry:
          Gear_D = 8;
        state Gear_1st
          entry:
          Gear_D = 1;
        state Gear_5th
          entry:
          Gear_D = 5;
        state Gear_2nd
          entry:
          Gear_D  = 2;
        (default) -> Gear_1st
        Gear_2nd -> Gear_3rd [order 1] : UP
        Gear_7th -> Gear_8th [order 1] : UP
        Gear_4th -> Gear_5th [order 1] : UP
        Gear_5th -> Gear_6th [order 1] : UP
        Gear_6th -> Gear_7th [order 1] : UP
        Gear_3rd -> Gear_4th [order 1] : UP
        Gear_1st -> Gear_2nd : UP
        Gear_3rd -> Gear_2nd [order 2] : DOWN
        Gear_4th -> Gear_3rd [order 2] : DOWN
        Gear_2nd -> Gear_1st [order 2] : DOWN
        Gear_5th -> Gear_4th [order 2] : DOWN
        Gear_6th -> Gear_5th [order 2] : DOWN
        Gear_7th -> Gear_6th [order 2] : DOWN
        Gear_8th -> Gear_7th : DOWN
      state Gear_Transient_D [parallel]
        du:[up_thrsh]=calc_up(Gear_D, drvAPP);
        du:[down_thrsh]=calc_down(Gear_D, drvAPP);
        settings: executionOrder=2
        state steady_state
        state upshifting
        state downshifting
        (default) -> steady_state
        steady_state -> upshifting [order 1] : [VehicleSpeed > up_thrsh && Gear_D < 8]
        steady_state -> downshifting [order 2] : [VehicleSpeed < down_thrsh && Gear_D > 1]
        downshifting -> steady_state [order 2] : [VehicleSpeed > down_thrsh]
        downshifting -> steady_state [order 1] : after(0.1,sec)
            | [VehicleSpeed <= down_thrsh]
            | {Gear_State_D.DOWN;}
        upshifting -> steady_state [order 1] : after(0.1,sec)
            | [VehicleSpeed >= up_thrsh]
            | {Gear_State_D.UP;}
        upshifting -> steady_state [order 2] : [VehicleSpeed < up_thrsh]
      state PlotShiftSchedule [function]
      state up_th = calc_up(Gear, APP) [function]
      state down_th = calc_down(Gear, APP) [function]
  data: Gear function_input; APP function_input; lockup_th function_output; Gear function_input; APP function_input; unlock_th function_output; Gear function_input; APP function_input; up_th function_output; Gear function_input; APP function_input; down_th function_output; tc_lockup_thrsh input double; Gear_D local int8 =1; drvAPP input double [0..100]; VehicleSpeed input double; TransEstGear output int8; down_thrsh local double =0; up_thrsh local double =0; LockupCmd output boolean; tc_spd_in input double; tc_spd_out input double; drvBPP input double; ShftLvrPos input int8; lockup_thrsh local double; unlock_thrsh local double
  events: DOWN local EITHER_EDGE_EVENT; UP local EITHER_EDGE_EVENT

== stateflow chart Hybrid_P2_Parallel_ETE/Controller_with_Transmission_Manager1/HSC/Camaro Fault Detection/Component Diagnostic/Transmission Component Diagnostic/TCM_CompDia ==
  state TCM_Offline
    en: TCM_Status=0;
  state TCM_Limited [commented out]
    en: TCM_Status=1;
  state TCM_Online
    en: TCM_Status=2;
  (default) -> TCM_Offline
  TCM_Online -> TCM_Offline : [~TCMRollingAliveActive_SigValid||...
      | ~LvrPosTrnsShft_SigValid||...
      | ~TransEstGear_SigValid||...
      | ~LockupCmd_SigValid||VehDirFault]
  TCM_Offline -> TCM_Online : [TCMRollingAliveActive_SigValid&&...
      | LvrPosTrnsShft_SigValid&&TransEstGear_SigValid&&...
      | LockupCmd_SigValid&&VehDirFault==0]
  TCM_Online -> TCM_Limited [commented out]
  TCM_Limited -> TCM_Online [commented out]
  data: TCM_Status output; TCMRollingAliveActive_SigValid input; LvrPosTrnsShft_SigValid input; TransEstGear_SigValid input; LockupCmd_SigValid input; VehDirFault input

== stateflow chart Hybrid_P2_Parallel_ETE/Controller_with_Transmission_Manager1/HSC/Camaro Fault Detection/Input Conversions/TCM_Conversions/TCM_RollinAliveCounter/Rolling Alive Counter1 ==
  state RollingAliveCounter
    state Count1
      en: RollingAliveCnt=0;
    state Count2
      en: RollingAliveCnt=1;
    state Count3
      en: RollingAliveCnt=2;
    state Count4
      en: RollingAliveCnt=3;
    (default) -> Count1
    Count4 -> Count1 : after(0.01,sec)
    Count1 -> Count2 : after(0.01,sec)
    Count2 -> Count3 : after(0.01,sec)
    Count3 -> Count4 : after(0.01,sec)
  data: RollingAliveCnt output double

== stateflow chart Hybrid_P2_Parallel_ETE/Controller_with_Transmission_Manager1/HSC/Camaro Fault Detection/Signal Diagnostic/Engine Signal Diagnostic/Engine_Temp[DegC] ==
  state AboveMax
    en: EngTempRange=3;
  state HighRange
    en: EngTempRange=2;
  state NormalRange
    en: EngTempRange=1;
  HighRange -> AboveMax [order 2] : [Engine_Temp_DegC>120]
  AboveMax -> HighRange : [Engine_Temp_DegC<120]
  NormalRange -> HighRange [order 1] : [Engine_Temp_DegC>100&&Engine_Temp_DegC<120]
  HighRange -> NormalRange [order 1] : [Engine_Temp_DegC<=100]
  NormalRange -> NormalRange [order 2] : [clearFaults==1]
      | {EngTempRange=1;}
  (default) -> NormalRange
  data: clearFaults input; Engine_Temp_DegC input; EngTempRange output; data local
